simulink model "Sim_Uncertain_CDelay_simtest"  (Simulink 7.3)
settings: Solver=VariableStepDiscrete  StartTime=0.0  StopTime=10  FixedStep=1e-10  RelTol=1e-3
settings Model: Creator=MD710  LastModifiedBy=MD710
settings DebuggingCC: SaveWithParameterizedLinksMsg=none  SolverPrmCheckMsg=none  MultiTaskDSMMsg=warning  MultiTaskCondExecSysMsg=none  FcnCallInpInsideContextMsg=Enable All  StrictBusMsg=None
settings HardwareCC: TargetHWDeviceType=32-bit Generic
settings RTWCC: IncludeERTFirstTime=on
settings GRTTargetCC: TargetFcnLib=ansi_tfl_tmw.mat

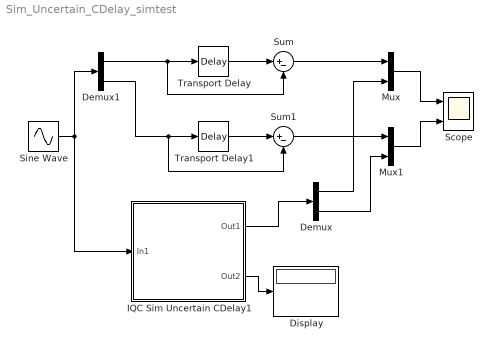
== system Sim_Uncertain_CDelay_simtest ==
  Demux : Demux  Outputs=2
  Demux1 : Demux  Outputs=2
  Display : Display
  IQC Sim Uncertain CDelay1 : Subsystem  mask(IQC Sim Uncertain CDelay(ver:0.1)){sou_del=Custom, max_del=1, num_ran=1, cus=[0.3 0.8], iqc1=on, iqc1_pole=[], iqc1_out='', iqc2=off, lis_rel='', delay_time=0}
      mask prompts: sou_del "Source of the delay:(Default: Random)"; max_del "Maximum Delay:"; num_ran "The Number of Random:(1 or input_dim)"; cus "Custom:"; iqc1 "iqc_cdelay(Input,Maximum Delay,Pole)"; iqc1_pole "Pole:(Default: [])"; iqc1_out "Output Variable:(Default: empty)"; iqc2 "Custom IQC"; lis_rel "List of IQC Relationships:"; delay_time "Mask Parameter 10:"
      mask init:
      | switch sou_del
      |     case 1
      |         delay_time=max_del*rand(1,num_ran);
      |     case 2
      |         delay_time=reshape(cus,1,length(cus));
      | end
      | % fprintf('The Random Delay Time: %4.3f \n',delay_time);
      mask Help: <a href="matlab:doc iqc_cdelay;">iqc_cdelay</a>
      mask StyleString: popup(Random|Custom),edit,edit,edit,checkbox,edit,edit,checkbox,edit,edit
      mask CallbackString: iqc_block_cho(gcb,'sim_uncertaincdelay_sou')||||iqc_block_cho(gcb,'sim_uncertaincdelay_iqc1')|||iqc_block_cho(gcb,'sim_uncertaincdelay_iqc2')||
      mask TabNameString: Simulink Parameters,Simulink Parameters,Simulink Parameters,Simulink Parameters,Procedure Parameters,Procedure Parameters,Procedure Parameters,Procedure Parameters,Procedure Parameters,Simulink Parameters
      mask Display: disp('\fontsize{14}exp(-T*s)-1', 'texmode','on');port_label('input',1,'in');port_label('output',1,'out');port_label('output',2,'T');
  Mux : Mux  Inputs=2
  Mux1 : Mux  Inputs=2
  Scope : Scope  NumInputPorts=2
      settings: YMin=-5~-5  YMax=5~5
  Sine Wave : Sin  Amplitude=[1.1 2.2]  Bias=[0 0]  Frequency=[1 1]  Phase=[0 0]  Samples=10  SampleTime=[0 0]  Offset=0
  Sum : Sum  Inputs=|+-
  Sum1 : Sum  Inputs=|+-
  Transport Delay : TransportDelay  DelayTime=0.3
  Transport Delay1 : TransportDelay  DelayTime=0.8
  wires:
  Sine Wave/1 -> IQC Sim Uncertain CDelay1/1(In1), Demux1/1
  IQC Sim Uncertain CDelay1/2(Out2) -> Display/1
  IQC Sim Uncertain CDelay1/1(Out1) -> Demux/1
  Transport Delay/1 -> Sum/1
  Transport Delay1/1 -> Sum1/1
  Sum/1 -> Mux/1
  Demux/1 -> Mux/2
  Sum1/1 -> Mux1/1
  Demux/2 -> Mux1/2
  Mux/1 -> Scope/1
  Mux1/1 -> Scope/2
  Demux1/1 -> Transport Delay/1, Sum/2
  Demux1/2 -> Sum1/2, Transport Delay1/1

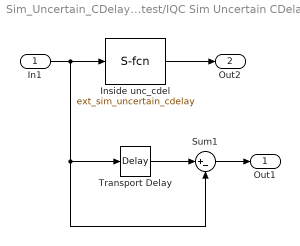
== system Sim_Uncertain_CDelay_simtest/IQC Sim Uncertain CDelay1 ==
  In1 : Inport
  Inside unc_cdel : M-S-Function  FunctionName=ext_sim_uncertain_cdelay  Parameters=sou_del,max_del,num_ran,cus,iqc1,iqc1_pole,iqc1_out,iqc2,lis_rel,delay_time
  Sum1 : Sum  Inputs=|+-
  Transport Delay : TransportDelay  DelayTime=delay_time
  Out1 : Outport
  Out2 : Outport  Port=2
  wires:
  Sum1/1 -> Out1/1
  In1/1 -> Sum1/2, Transport Delay/1, Inside unc_cdel/1
  Transport Delay/1 -> Sum1/1
  Inside unc_cdel/1 -> Out2/1
